simulink model "AION_request_fail_analysis"  (R2021a)
settings: configuration reference "AION_IDS_Speedgoat" (kept outside this file)
settings Model: DataDictionary=AION_request_fail_analysis.sldd  Creator=Administrator  LastModifiedBy=Administrator
settings ConfigSetRef: SourceName=AION_IDS_Speedgoat

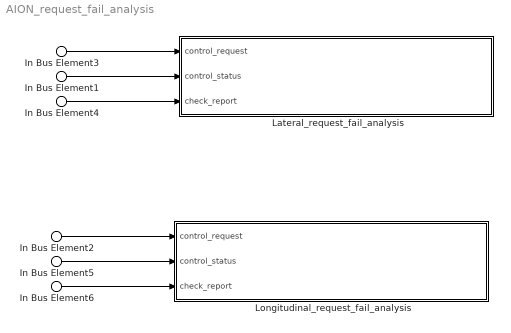
== system AION_request_fail_analysis ==
  In Bus Element3 : Inport  PortName=InBus  Element=set_lateral_control_info.set_LatCtrlReq
  In Bus Element2 : Inport  PortName=InBus  Element=set_longitudinal_control_info.set_LngCtrlReq
  In Bus Element4 : Inport  PortName=InBus  Element=get_SCU_info.get_LatAutoCheckReport
  In Bus Element1 : Inport  PortName=InBus  Element=get_SCU_info.get_LatCtrlMode
  In Bus Element6 : Inport  PortName=InBus  Element=get_SCU_info.get_LngAutoCheckIReport
  In Bus Element5 : Inport  PortName=InBus  Element=get_SCU_info.get_LngCtrlMode
  Lateral_request_fail_analysis : MATLAB Function  TreatAsAtomicUnit=on
  Longitudinal_request_fail_analysis : MATLAB Function  TreatAsAtomicUnit=on
  wires:
  In Bus Element4/1 -> Lateral_request_fail_analysis/3(check_report)
  In Bus Element3/1 -> Lateral_request_fail_analysis/1(control_request)
  In Bus Element1/1 -> Lateral_request_fail_analysis/2(control_status)
  In Bus Element6/1 -> Longitudinal_request_fail_analysis/3(check_report)
  In Bus Element2/1 -> Longitudinal_request_fail_analysis/1(control_request)
  In Bus Element5/1 -> Longitudinal_request_fail_analysis/2(control_status)

== matlab function AION_request_fail_analysis/Longitudinal_request_fail_analysis ==
  data: control_request input; control_status input Enum: Control_status size=1; check_report input
% 操作模式判断
function longitudinal_request_fail_analysis(control_request,control_status,check_report)
%   1.输入参数：
%       (1)control_request           横向控制请求
%       (2)control_status            横向控制功能状态
%       (3)check_report              检查报告记录
%   2.输出参数：
%       无

%% 静态变量声明及初始化
% 请求失败计数
persistent request_fail_count
if isempty(request_fail_count)
   request_fail_count = 0;
end
%%
    if((control_request == Control_request.Auto)&&(control_status == Control_status.ManualStatus))
        request_fail_count = request_fail_count + 1; 
    else 
        request_fail_count = 0;
    end    
    if request_fail_count > 2
        if(bitand(check_report,0x00000000) == 0x00000000)
           disp('Lng_req_fail Bit0 Fault');
        end
        if(bitand(check_report,0x00000001) == 0x00000001)
           disp('Lng_req_fail Bit1 Fault');
        end
        if(bitand(check_report,0x00000002) == 0x00000002)
           disp('Lng_req_fail Bit2 Fault');
        end
        if(bitand(check_report,0x00000004) == 0x00000004)
           disp('Lng_req_fail Bit3 Fault');
        end
        if(bitand(check_report,0x00000008) == 0x00000008)
           disp('Lng_req_fail Bit4 Fault');
        end
        if(bitand(check_report,0x00000010) == 0x00000010)
           disp('Lng_req_fail Bit5 Fault');
        end
        if(bitand(check_report,0x00000020) == 0x00000020)
           disp('Lng_req_fail Bit6 Fault');
        end
        if(bitand(check_report,0x00000040) == 0x00000040)
           disp('Lng_req_fail Bit7 Fault');
        end
        if(bitand(check_report,0x00000080) == 0x00000080)
           disp('Lng_req_fail Bit8 Fault');
        end
        if(bitand(check_report,0x00000100) == 0x00000100)
           disp('Lng_req_fail Bit9 Fault');
        end
        if(bitand(check_report,0x00000200) == 0x00000200)
           disp('Lng_req_fail Bit10 Fault');
        end
        if(bitand(check_report,0x00000400) == 0x00000400)
           disp('Lng_req_fail Bit11 Fault');
        end
        if(bitand(check_report,0x00000800) == 0x00000800)
           disp('Lng_req_fail Bit12 Fault');
        end
        if(bitand(check_report,0x00001000) == 0x00001000)
           disp('Lng_req_fail Bit13 Fault');
        end
    end
end

== matlab function AION_request_fail_analysis/Lateral_request_fail_analysis ==
  data: control_request input; control_status input Enum: Control_status size=1; check_report input
% 操作模式判断
function lateral_request_fail_analysis(control_request,control_status,check_report)
%   1.输入参数：
%       (1)control_request           横向控制请求
%       (2)control_status            横向控制功能状态
%       (3)check_report              检查报告记录
%   2.输出参数：
%       无

%% 静态变量声明及初始化
% 请求失败计数
persistent request_fail_count
if isempty(request_fail_count)
   request_fail_count = 0;
end
%%
    if((control_request == Control_request.Auto)&&(control_status == Control_status.ManualStatus))
        request_fail_count = request_fail_count + 1; 
    else 
        request_fail_count = 0;
    end    
    if request_fail_count > 2
        if(bitand(check_report,0x00000000) == 0x00000000)
           disp('Lat_req_fail Bit 0 Fault');
        end
        if(bitand(check_report,0x00000001) == 0x00000001)
           disp('Lat_req_fail Bit1 Fault');
        end
        if(bitand(check_report,0x00000002) == 0x00000002)
           disp('Lat_req_fail Bit2 Fault');
        end
        if(bitand(check_report,0x00000003) == 0x00000003)
           disp('Lat_req_fail Bit3 Fault');
        end
    end
end
